simulink model "c5mqft"  (R2019b)
settings: Solver=ode15s  StartTime=0.0  StopTime=1000  RelTol=1e-6
PreLoadFcn:
  | s=tf('s');
  | G=1.8393*0.0011^0.96/(1+s/0.29)^2*3.13*exp(-5*s)/(433.33*s+1);
  | ww=[1e-3 1e3]; N=5;
libraries: cstblocks x4
settings Model: Creator=xuedi  LastModifiedBy=xuedi
settings DataIOCC: SaveFormat=Array  ReturnWorkspaceOutputs=off
settings DebuggingCC: UnconnectedInputMsg=none  UnconnectedOutputMsg=none  UnconnectedLineMsg=none  SFMachineParentedDataDiag=error

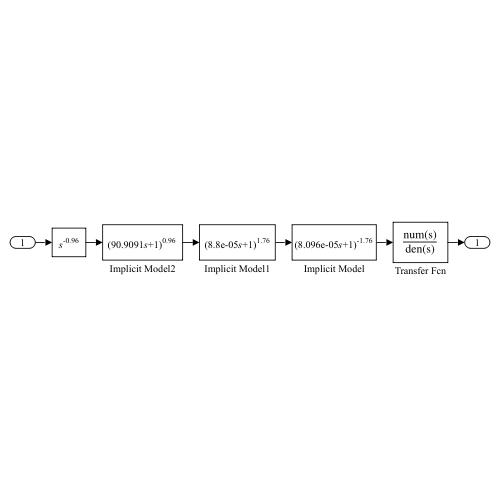
[thumbnail: Simulink's stored preview of the top-level diagram]
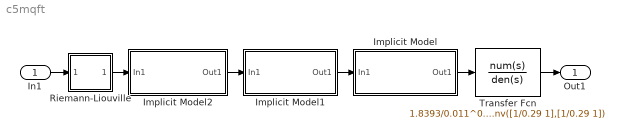
== system c5mqft ==
  In1 : Inport
  Implicit Model : Subsystem  mask{tau=8.096e-5, nu=1.76, ww=ww, N=N, keyCD=Continous}
      mask prompts: tau "Time constant tau"; nu "power nu"; ww "Frequency range [wb,wh]"; N "Filter order"; keyCD "Filter type"
      mask init:
      | str=['(' num2str(tau) '{\its}+1)^{' num2str(-nu) '}'];
      |    if keyCD==1, G=tf(1,1);
      |    else, T=ww(1); G=irid_folpf(tau,nu,T,N); end
      mask TypeOptions keyCD: Continous | Discrete Filter
      mask Display: disp(str,'texmode','on')
  Implicit Model1 : Subsystem  mask{tau=8.8e-5, nu=-1.76, ww=ww, N=N, keyCD=Continous}
      mask prompts: tau "Time constant tau"; nu "power nu"; ww "Frequency range [wb,wh]"; N "Filter order"; keyCD "Filter type"
      mask init:
      | str=['(' num2str(tau) '{\its}+1)^{' num2str(-nu) '}'];
      |    if keyCD==1, G=tf(1,1);
      |    else, T=ww(1); G=irid_folpf(tau,nu,T,N); end
      mask TypeOptions keyCD: Continous | Discrete Filter
      mask Display: disp(str,'texmode','on')
  Implicit Model2 : Subsystem  mask{tau=1/0.011, nu=-0.96, ww=ww, N=N, keyCD=Continous}
      mask prompts: tau "Time constant tau"; nu "power nu"; ww "Frequency range [wb,wh]"; N "Filter order"; keyCD "Filter type"
      mask init:
      | str=['(' num2str(tau) '{\its}+1)^{' num2str(-nu) '}'];
      |    if keyCD==1, G=tf(1,1);
      |    else, T=ww(1); G=irid_folpf(tau,nu,T,N); end
      mask TypeOptions keyCD: Continous | Discrete Filter
      mask Display: disp(str,'texmode','on')
  "Riemann-Liouville " : Subsystem  mask{gam=-0.96, ww=ww, n=N, kF1=off, kF=Oustaloup filter}
      mask prompts: gam "Derivative order gamma"; ww "Frequency range [wb,wh]"; n "Apprixmation order"; kF1 "Is a low-pass filter required?"; kF "Filter type"
      mask init:
      | wb=ww(1); wh=ww(2); 
      | if isnumeric(gam), str=['{\its}^{' num2str(gam) '}']; 
      | else, str='{\its}^{\gamma}'; end
      | if kF==1, G=ousta_fod(gam,n,wb,wh);
      | elseif kF==2, G=new_fod(gam,n,wb,wh); 
      | else, G=matsuda_fod(gam,n,wb,wh); end
      | T=1/wh; if kF1==1, G=G*tf(1,[T 1]); end
      mask TypeOptions kF: Oustaloup filter | Modified Oustaloup filter | Matsuda-Fujii filter
      mask Display: disp(str,'texmode','on')
  Transfer Fcn : TransferFcn  Numerator=1.8393/0.011^0.96  Denominator=conv([1/0.29 1],[1/0.29 1])
  Out1 : Outport
  wires:
  Implicit Model2/1(Out1) -> Implicit Model1/1(In1)
  Implicit Model1/1(Out1) -> Implicit Model/1(In1)
  In1/1 -> "Riemann-Liouville "/1(In1)
  "Riemann-Liouville "/1(Out1) -> Implicit Model2/1(In1)
  Transfer Fcn/1 -> Out1/1
  Implicit Model/1(Out1) -> Transfer Fcn/1

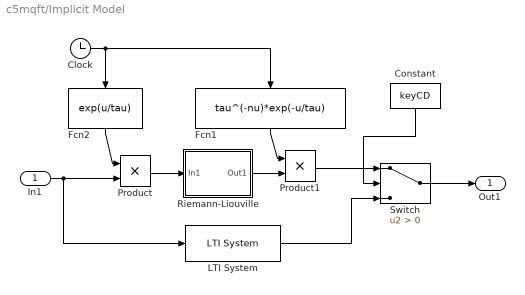
== system c5mqft/Implicit Model ==
  In1 : Inport
  Clock : Clock
  Constant : Constant  Value=keyCD
  Fcn1 : Fcn  Expr=tau^(-nu)*exp(-u/tau)
  Fcn2 : Fcn  Expr=exp(u/tau)
  LTI System : cstblocks/LTI System  sys=G  IC=[]
  Product : Product
  Product1 : Product
  "Riemann-Liouville " : Subsystem  mask{gam=-nu, ww=ww, n=N, kF1=on, kF=Oustaloup filter}
      mask prompts: gam "Derivative order gamma"; ww "Frequency range [wb,wh]"; n "Apprixmation order"; kF1 "Is a low-pass filter required?"; kF "Filter type"
      mask init:
      | wb=ww(1); wh=ww(2); 
      | if kF==1, G=ousta_fod(gam,n,wb,wh);
      | else, G=new_fod(gam,n,wb,wh); end
      | G=tf(G); num=G.num{1}; den=G.den{1}; T=1/wh; 
      | if isnumeric(gam), str=['{\its}^{' num2str(gam) '}']; 
      | else, str='{\its}^{gam}'; end
      | if kF1==1, G=G*tf(1,[T 1]); end
      mask TypeOptions kF: Oustaloup filter | Modified Oustaloup filter | Matsuda-Fujii filter
      mask Display: disp(str,'texmode','on')
  Switch : Switch  Criteria=u2 > Threshold
  Out1 : Outport
  wires:
  Clock/1 -> Fcn1/1, Fcn2/1
  Fcn1/1 -> Product1/1
  "Riemann-Liouville "/1(Out1) -> Product1/2
  Product/1 -> "Riemann-Liouville "/1(In1)
  Fcn2/1 -> Product/1
  Product1/1 -> Switch/1
  Switch/1 -> Out1/1
  Constant/1 -> Switch/2
  In1/1 -> LTI System/1, Product/2
  LTI System/1 -> Switch/3

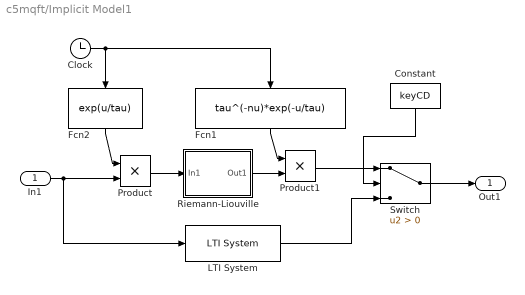
== system c5mqft/Implicit Model1 ==
  In1 : Inport
  Clock : Clock
  Constant : Constant  Value=keyCD
  Fcn1 : Fcn  Expr=tau^(-nu)*exp(-u/tau)
  Fcn2 : Fcn  Expr=exp(u/tau)
  LTI System : cstblocks/LTI System  sys=G  IC=[]
  Product : Product
  Product1 : Product
  "Riemann-Liouville " : Subsystem  mask{gam=-nu, ww=ww, n=N, kF1=on, kF=Oustaloup filter}
      mask prompts: gam "Derivative order gamma"; ww "Frequency range [wb,wh]"; n "Apprixmation order"; kF1 "Is a low-pass filter required?"; kF "Filter type"
      mask init: same as c5mqft/Implicit Model/Riemann-Liouville 
      mask TypeOptions kF: Oustaloup filter | Modified Oustaloup filter | Matsuda-Fujii filter
      mask Display: disp(str,'texmode','on')
  Switch : Switch  Criteria=u2 > Threshold
  Out1 : Outport
  wires:
  LTI System/1 -> Switch/3
  In1/1 -> Product/2, LTI System/1
  Constant/1 -> Switch/2
  Switch/1 -> Out1/1
  Product1/1 -> Switch/1
  Fcn2/1 -> Product/1
  Product/1 -> "Riemann-Liouville "/1(In1)
  "Riemann-Liouville "/1(Out1) -> Product1/2
  Fcn1/1 -> Product1/1
  Clock/1 -> Fcn2/1, Fcn1/1

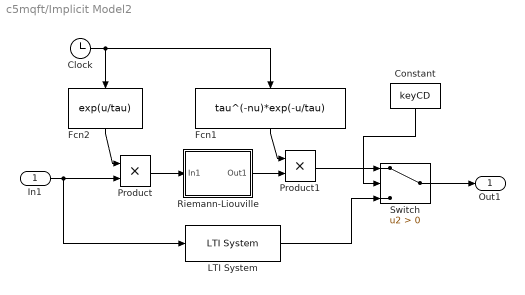
== system c5mqft/Implicit Model2 ==
  In1 : Inport
  Clock : Clock
  Constant : Constant  Value=keyCD
  Fcn1 : Fcn  Expr=tau^(-nu)*exp(-u/tau)
  Fcn2 : Fcn  Expr=exp(u/tau)
  LTI System : cstblocks/LTI System  sys=G  IC=[]
  Product : Product
  Product1 : Product
  "Riemann-Liouville " : Subsystem  mask{gam=-nu, ww=ww, n=N, kF1=on, kF=Oustaloup filter}
      mask prompts: gam "Derivative order gamma"; ww "Frequency range [wb,wh]"; n "Apprixmation order"; kF1 "Is a low-pass filter required?"; kF "Filter type"
      mask init: same as c5mqft/Implicit Model/Riemann-Liouville 
      mask TypeOptions kF: Oustaloup filter | Modified Oustaloup filter | Matsuda-Fujii filter
      mask Display: disp(str,'texmode','on')
  Switch : Switch  Criteria=u2 > Threshold
  Out1 : Outport
  wires:
  Clock/1 -> Fcn1/1, Fcn2/1
  Fcn1/1 -> Product1/1
  "Riemann-Liouville "/1(Out1) -> Product1/2
  Product/1 -> "Riemann-Liouville "/1(In1)
  Fcn2/1 -> Product/1
  Product1/1 -> Switch/1
  Switch/1 -> Out1/1
  Constant/1 -> Switch/2
  In1/1 -> LTI System/1, Product/2
  LTI System/1 -> Switch/3

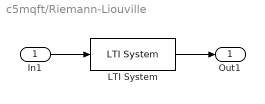
== system c5mqft/Riemann-Liouville  ==
  In1 : Inport
  LTI System : cstblocks/LTI System  sys=G  IC=[]
  Out1 : Outport
  wires:
  In1/1 -> LTI System/1
  LTI System/1 -> Out1/1

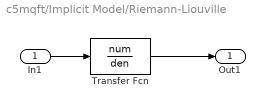
== system c5mqft/Implicit Model/Riemann-Liouville  ==
  In1 : Inport
  Transfer Fcn : TransferFcn  Numerator=num  Denominator=den
  Out1 : Outport
  wires:
  In1/1 -> Transfer Fcn/1
  Transfer Fcn/1 -> Out1/1

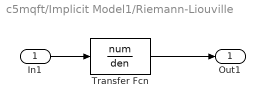
== system c5mqft/Implicit Model1/Riemann-Liouville  ==
  In1 : Inport
  Transfer Fcn : TransferFcn  Numerator=num  Denominator=den
  Out1 : Outport
  wires:
  Transfer Fcn/1 -> Out1/1
  In1/1 -> Transfer Fcn/1

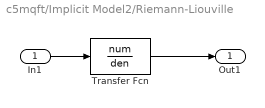
== system c5mqft/Implicit Model2/Riemann-Liouville  ==
  In1 : Inport
  Transfer Fcn : TransferFcn  Numerator=num  Denominator=den
  Out1 : Outport
  wires:
  In1/1 -> Transfer Fcn/1
  Transfer Fcn/1 -> Out1/1
